simulink model "TwoTankClosedLoop"  (R2016a)
settings: Solver=ode45  StartTime=0.0  StopTime=inputOpt.simTime  MaxStep=0.2  RelTol=1e-3
undefined symbols (not defined in the file): Initials, inputOpt, kl, kv1, kv2, kv3, kv4, L1i, SPL1, SPL2, SPT1, SPT2, T1i, timeDelay
libraries: simulink x4
settings Model: Creator=blindner  LastModifiedBy=blindner
settings DataIOCC: ExternalInput=getinputstruct(op_trim1)  FinalStateName=TwoTankClosedLoopSimState  InitialState=simState  SaveFinalState=on  SaveCompleteFinalSimState=on  SaveFormat=Array  SaveOutput=off  InspectSignalLogs=on  SaveTime=off
settings DebuggingCC: SolverPrmCheckMsg=warning
settings HardwareCC: ProdBitPerPointer=32  ProdLargestAtomicFloat=None  ProdIntDivRoundTo=Undefined  ProdEndianess=Unspecified  ProdWordSize=32  ProdHWDeviceType=32-bit Generic
settings ModelReferenceCC: PropagateSignalLabelsOutOfModel=off
settings ConfigComp: CovModelRefEnable=Off  CovSFcnEnable=off

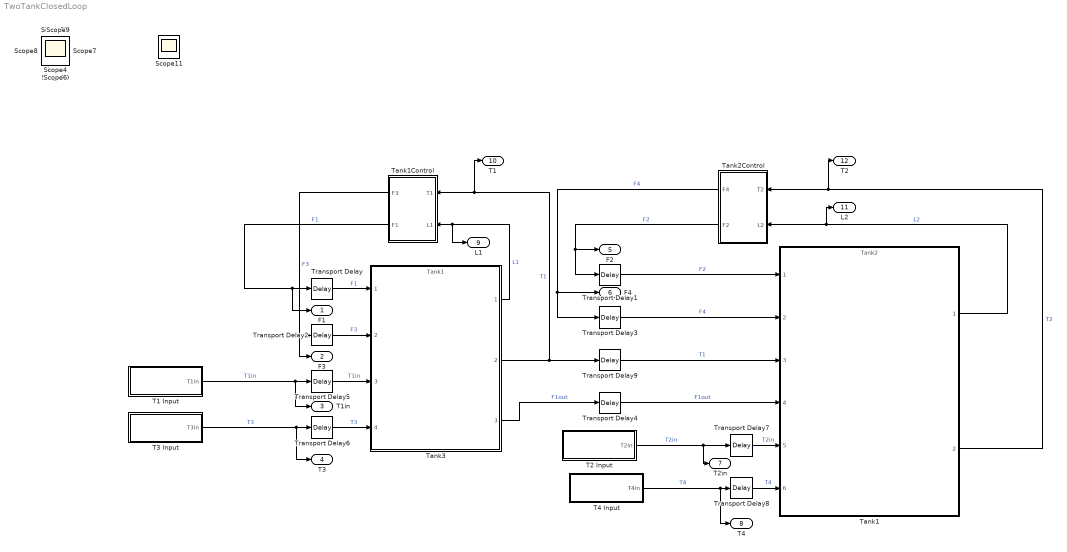
== system TwoTankClosedLoop ==
  T1 Input : Subsystem  Variant=on
  T2 Input : Subsystem  Variant=on
  T3 Input : Subsystem  Variant=on
  T4 Input : Subsystem  Variant=on
  Tank1 : ModelReference  ModelNameDialog=Tank2  SimulationMode=Normal  ModelReferenceVersion=1.153
  Tank1Control : Subsystem
  Tank2Control : Subsystem
  Tank3 : ModelReference  ModelNameDialog=Tank1  SimulationMode=Normal  ModelReferenceVersion=1.161
  Transport Delay : TransportDelay  DelayTime=timeDelay.F1  InitialOutput=Initials.F1  TransDelayFeedthrough=on
  Transport Delay1 : TransportDelay  DelayTime=timeDelay.F2  InitialOutput=Initials.F2  TransDelayFeedthrough=on
  Transport Delay2 : TransportDelay  DelayTime=timeDelay.F3  InitialOutput=Initials.F3  TransDelayFeedthrough=on
  Transport Delay3 : TransportDelay  DelayTime=timeDelay.F4  InitialOutput=Initials.F4  TransDelayFeedthrough=on
  Transport Delay4 : TransportDelay  DelayTime=timeDelay.F1Out  InitialOutput=(L1i)^0.5*kl  TransDelayFeedthrough=on
  Transport Delay5 : TransportDelay  DelayTime=timeDelay.F1  InitialOutput=inputOpt.T1in.start  TransDelayFeedthrough=on
  Transport Delay6 : TransportDelay  DelayTime=timeDelay.F3  InitialOutput=inputOpt.T3.start  TransDelayFeedthrough=on
  Transport Delay7 : TransportDelay  DelayTime=timeDelay.F2  InitialOutput=inputOpt.T2in.start  TransDelayFeedthrough=on
  Transport Delay8 : TransportDelay  DelayTime=timeDelay.F4  InitialOutput=inputOpt.T4.start  TransDelayFeedthrough=on
  Transport Delay9 : TransportDelay  DelayTime=timeDelay.F1Out  InitialOutput=T1i  TransDelayFeedthrough=on
  F1 : Outport
  F3 : Outport  Port=2
  T1in : Outport  Port=3
  T3 : Outport  Port=4
  F2 : Outport  Port=5
  F4 : Outport  Port=6
  T2in : Outport  Port=7
  T4 : Outport  Port=8
  L1 : Outport  Port=9
  T1 : Outport  Port=10
  L2 : Outport  Port=11
  T2 : Outport  Port=12
  Scope{,1..11} (12 alike) : Scope
  wires:
  Tank2Control/2(F2) -> Transport Delay1/1, F2/1  "F2"
  T2 Input/1(T2in) -> T2in/1, Transport Delay7/1  "T2in"
  Tank1/2 -> T2/1, Tank2Control/1(T2)  "T2"
  T1 Input/1(T1in) -> T1in/1, Transport Delay5/1  "T1in"
  T3 Input/1(T3in) -> T3/1, Transport Delay6/1  "T3"
  Tank1Control/2(F1) -> F1/1, Transport Delay/1  "F1"
  Tank3/3 -> Transport Delay4/1  "F1out"
  T4 Input/1(T4in) -> T4/1, Transport Delay8/1  "T4"
  Tank1Control/1(F3) -> F3/1, Transport Delay2/1  "F3"
  Tank2Control/1(F4) -> F4/1, Transport Delay3/1  "F4"
  Transport Delay5/1 -> Tank3/3  "T1in"
  Transport Delay6/1 -> Tank3/4  "T3"
  Transport Delay/1 -> Tank3/1  "F1"
  Transport Delay2/1 -> Tank3/2  "F3"
  Transport Delay3/1 -> Tank1/2  "F4"
  Transport Delay8/1 -> Tank1/6  "T4"
  Transport Delay7/1 -> Tank1/5  "T2in"
  Transport Delay9/1 -> Tank1/3  "T1"
  Transport Delay4/1 -> Tank1/4  "F1out"
  Transport Delay1/1 -> Tank1/1  "F2"
  Tank3/2 -> T1/1, Tank1Control/1(T1), Transport Delay9/1  "T1"
  Tank1/1 -> L2/1, Tank2Control/2(L2)  "L2"
  Tank3/1 -> L1/1, Tank1Control/2(L1)  "L1"

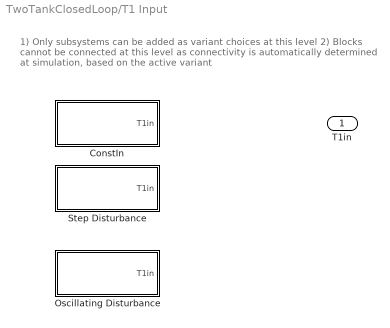
== system TwoTankClosedLoop/T1 Input ==
  note: 1) Only subsystems can be added as variant choices at this level
      | 2) Blocks cannot be connected at this level as connectivity is
      | automatically determined at simulation, based on the active variant
  ConstIn : Subsystem  VariantControl=(default)
  Oscillating Disturbance : Subsystem  VariantControl=T1Oscillating
  Step Disturbance : Subsystem  VariantControl=T1Step
  T1in : Outport

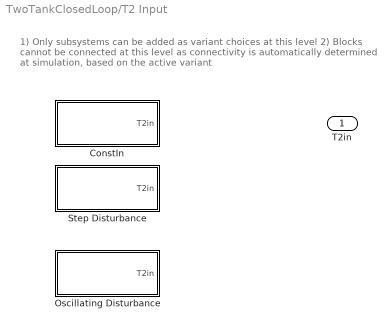
== system TwoTankClosedLoop/T2 Input ==
  note: 1) Only subsystems can be added as variant choices at this level
      | 2) Blocks cannot be connected at this level as connectivity is
      | automatically determined at simulation, based on the active variant
  ConstIn : Subsystem  VariantControl=(default)
  Oscillating Disturbance : Subsystem  VariantControl=T2Oscillating
  Step Disturbance : Subsystem  VariantControl=T2Step
  T2in : Outport

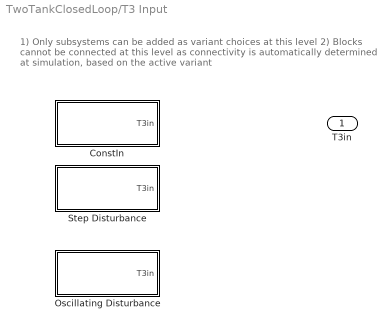
== system TwoTankClosedLoop/T3 Input ==
  note: 1) Only subsystems can be added as variant choices at this level
      | 2) Blocks cannot be connected at this level as connectivity is
      | automatically determined at simulation, based on the active variant
  ConstIn : Subsystem  VariantControl=(default)
  Oscillating Disturbance : Subsystem  VariantControl=T3Oscillating
  Step Disturbance : Subsystem  VariantControl=T3Step
  T3in : Outport

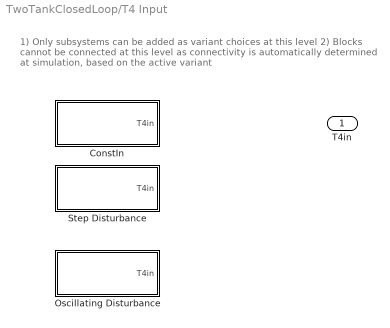
== system TwoTankClosedLoop/T4 Input ==
  note: 1) Only subsystems can be added as variant choices at this level
      | 2) Blocks cannot be connected at this level as connectivity is
      | automatically determined at simulation, based on the active variant
  ConstIn : Subsystem  VariantControl=(default)
  Oscillating Disturbance : Subsystem  VariantControl=T4Oscillating
  Step Disturbance : Subsystem  VariantControl=T4Step
  T4in : Outport

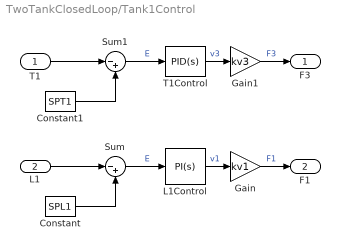
== system TwoTankClosedLoop/Tank1Control ==
  T1 : Inport
  L1 : Inport  Port=2
  Constant : Constant  Value=SPL1
  Constant1 : Constant  Value=SPT1
  Gain : Gain  Gain=kv1
  Gain1 : Gain  Gain=kv3
  L1Control : simulink/Continuous/PID Controller  Controller=PI  TimeDomain=Continuous-time  SampleTime=-1  IntegratorMethod=Forward Euler  FilterMethod=Forward Euler  Form=Parallel  UseFilter=on  ControllerParametersSource=internal  P=13  I=2  D=-46.1324731979825  N=0.0805995619975817  InitialConditionSource=internal  InitialConditionForIntegrator=Initials.F1/kv1  InitialConditionForFilter=0  ExternalReset=none  LimitOutput=on  UpperSaturationLimit=inf  LowerSaturationLimit=0  LinearizeAsGain=on  AntiWindupMode=none  Kb=1  TrackingMode=off  Kt=1  PParamMin=[]  PParamMax=[]  IParamMin=[]  IParamMax=[]  DParamMin=[]  DParamMax=[]  NParamMin=[]  NParamMax=[]  KbParamMin=[]  KbParamMax=[]  KtParamMin=[]  KtParamMax=[]  POutMin=[]  POutMax=[]  IOutMin=[]  IOutMax=[]  DOutMin=[]  DOutMax=[]  NOutMin=[]  NOutMax=[]  KbOutMin=[]  KbOutMax=[]  KtOutMin=[]  KtOutMax=[]  IntegratorOutMin=[]  IntegratorOutMax=[]  FilterOutMin=[]  FilterOutMax=[]  SumOutMin=[]  SumOutMax=[]  SumI1OutMin=[]  SumI1OutMax=[]  SumI2OutMin=[]  SumI2OutMax=[]  SumI3OutMin=[]  SumI3OutMax=[]  SumDOutMin=[]  SumDOutMax=[]  SaturationOutMin=[]  SaturationOutMax=[]  IntegratorContinuousStateAttributes=''  IntegratorStateMustResolveToSignalObject=off  IntegratorRTWStateStorageClass=Auto  FilterContinuousStateAttributes=''  FilterStateMustResolveToSignalObject=off  FilterRTWStateStorageClass=Auto  DifferentiatorICPrevScaledInput=0  DifferentiatorOutMin=[]  DifferentiatorOutMax=[]
  Sum : Sum  Inputs=|-+
  Sum1 : Sum  Inputs=|-+
  T1Control : simulink/Continuous/PID Controller  Controller=PID  TimeDomain=Continuous-time  SampleTime=-1  IntegratorMethod=Forward Euler  FilterMethod=Forward Euler  Form=Parallel  UseFilter=on  ControllerParametersSource=internal  P=9.53922380214598  I=1.41929760465604  D=0  N=100  InitialConditionSource=internal  InitialConditionForIntegrator=Initials.F3/kv3  InitialConditionForFilter=0  ExternalReset=none  LimitOutput=on  UpperSaturationLimit=inf  LowerSaturationLimit=0  LinearizeAsGain=on  AntiWindupMode=none  Kb=1  TrackingMode=off  Kt=1  PParamMin=[]  PParamMax=[]  IParamMin=[]  IParamMax=[]  DParamMin=[]  DParamMax=[]  NParamMin=[]  NParamMax=[]  KbParamMin=[]  KbParamMax=[]  KtParamMin=[]  KtParamMax=[]  POutMin=[]  POutMax=[]  IOutMin=[]  IOutMax=[]  DOutMin=[]  DOutMax=[]  NOutMin=[]  NOutMax=[]  KbOutMin=[]  KbOutMax=[]  KtOutMin=[]  KtOutMax=[]  IntegratorOutMin=[]  IntegratorOutMax=[]  FilterOutMin=[]  FilterOutMax=[]  SumOutMin=[]  SumOutMax=[]  SumI1OutMin=[]  SumI1OutMax=[]  SumI2OutMin=[]  SumI2OutMax=[]  SumI3OutMin=[]  SumI3OutMax=[]  SumDOutMin=[]  SumDOutMax=[]  SaturationOutMin=[]  SaturationOutMax=[]  IntegratorContinuousStateAttributes=''  IntegratorStateMustResolveToSignalObject=off  IntegratorRTWStateStorageClass=Auto  FilterContinuousStateAttributes=''  FilterStateMustResolveToSignalObject=off  FilterRTWStateStorageClass=Auto  DifferentiatorICPrevScaledInput=0  DifferentiatorOutMin=[]  DifferentiatorOutMax=[]
  F3 : Outport
  F1 : Outport  Port=2
  wires:
  Gain1/1 -> F3/1  "F3"
  Gain/1 -> F1/1  "F1"
  Sum1/1 -> T1Control/1  "E"
  Sum/1 -> L1Control/1  "E"
  T1Control/1 -> Gain1/1  "v3"
  L1Control/1 -> Gain/1  "v1"
  Constant1/1 -> Sum1/2
  Constant/1 -> Sum/2
  T1/1 -> Sum1/1
  L1/1 -> Sum/1

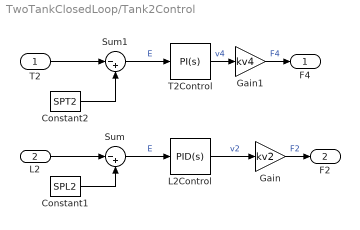
== system TwoTankClosedLoop/Tank2Control ==
  T2 : Inport
  L2 : Inport  Port=2
  Constant1 : Constant  Value=SPL2
  Constant2 : Constant  Value=SPT2
  Gain : Gain  Gain=kv2
  Gain1 : Gain  Gain=kv4
  L2Control : simulink/Continuous/PID Controller  Controller=PID  TimeDomain=Continuous-time  SampleTime=-1  IntegratorMethod=Forward Euler  FilterMethod=Forward Euler  Form=Parallel  UseFilter=on  ControllerParametersSource=internal  P=15  I=3  D=0  N=100  InitialConditionSource=internal  InitialConditionForIntegrator=Initials.F2/kv2  InitialConditionForFilter=0  ExternalReset=none  LimitOutput=on  UpperSaturationLimit=inf  LowerSaturationLimit=0  LinearizeAsGain=on  AntiWindupMode=none  Kb=1  TrackingMode=off  Kt=1  PParamMin=[]  PParamMax=[]  IParamMin=[]  IParamMax=[]  DParamMin=[]  DParamMax=[]  NParamMin=[]  NParamMax=[]  KbParamMin=[]  KbParamMax=[]  KtParamMin=[]  KtParamMax=[]  POutMin=[]  POutMax=[]  IOutMin=[]  IOutMax=[]  DOutMin=[]  DOutMax=[]  NOutMin=[]  NOutMax=[]  KbOutMin=[]  KbOutMax=[]  KtOutMin=[]  KtOutMax=[]  IntegratorOutMin=[]  IntegratorOutMax=[]  FilterOutMin=[]  FilterOutMax=[]  SumOutMin=[]  SumOutMax=[]  SumI1OutMin=[]  SumI1OutMax=[]  SumI2OutMin=[]  SumI2OutMax=[]  SumI3OutMin=[]  SumI3OutMax=[]  SumDOutMin=[]  SumDOutMax=[]  SaturationOutMin=[]  SaturationOutMax=[]  IntegratorContinuousStateAttributes=''  IntegratorStateMustResolveToSignalObject=off  IntegratorRTWStateStorageClass=Auto  FilterContinuousStateAttributes=''  FilterStateMustResolveToSignalObject=off  FilterRTWStateStorageClass=Auto  DifferentiatorICPrevScaledInput=0  DifferentiatorOutMin=[]  DifferentiatorOutMax=[]
  Sum : Sum  Inputs=|-+
  Sum1 : Sum  Inputs=|-+
  T2Control : simulink/Continuous/PID Controller  Controller=PI  TimeDomain=Continuous-time  SampleTime=-1  IntegratorMethod=Forward Euler  FilterMethod=Forward Euler  Form=Parallel  UseFilter=on  ControllerParametersSource=internal  P=5  I=0.5  D=0  N=100  InitialConditionSource=internal  InitialConditionForIntegrator=Initials.F4/kv4  InitialConditionForFilter=0  ExternalReset=none  LimitOutput=on  UpperSaturationLimit=inf  LowerSaturationLimit=0  LinearizeAsGain=on  AntiWindupMode=none  Kb=1  TrackingMode=off  Kt=1  PParamMin=[]  PParamMax=[]  IParamMin=[]  IParamMax=[]  DParamMin=[]  DParamMax=[]  NParamMin=[]  NParamMax=[]  KbParamMin=[]  KbParamMax=[]  KtParamMin=[]  KtParamMax=[]  POutMin=[]  POutMax=[]  IOutMin=[]  IOutMax=[]  DOutMin=[]  DOutMax=[]  NOutMin=[]  NOutMax=[]  KbOutMin=[]  KbOutMax=[]  KtOutMin=[]  KtOutMax=[]  IntegratorOutMin=[]  IntegratorOutMax=[]  FilterOutMin=[]  FilterOutMax=[]  SumOutMin=[]  SumOutMax=[]  SumI1OutMin=[]  SumI1OutMax=[]  SumI2OutMin=[]  SumI2OutMax=[]  SumI3OutMin=[]  SumI3OutMax=[]  SumDOutMin=[]  SumDOutMax=[]  SaturationOutMin=[]  SaturationOutMax=[]  IntegratorContinuousStateAttributes=''  IntegratorStateMustResolveToSignalObject=off  IntegratorRTWStateStorageClass=Auto  FilterContinuousStateAttributes=''  FilterStateMustResolveToSignalObject=off  FilterRTWStateStorageClass=Auto  DifferentiatorICPrevScaledInput=0  DifferentiatorOutMin=[]  DifferentiatorOutMax=[]
  F4 : Outport
  F2 : Outport  Port=2
  wires:
  Gain1/1 -> F4/1  "F4"
  Gain/1 -> F2/1  "F2"
  Sum1/1 -> T2Control/1  "E"
  Sum/1 -> L2Control/1  "E"
  Constant1/1 -> Sum/2
  Constant2/1 -> Sum1/2
  L2Control/1 -> Gain/1  "v2"
  T2Control/1 -> Gain1/1  "v4"
  T2/1 -> Sum1/1
  L2/1 -> Sum/1

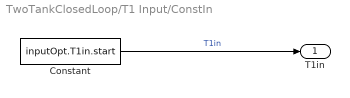
== system TwoTankClosedLoop/T1 Input/ConstIn ==
  Constant : Constant  Value=inputOpt.T1in.start
  T1in : Outport
  wires:
  Constant/1 -> T1in/1  "T1in"

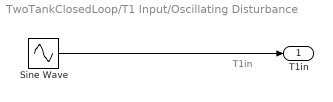
== system TwoTankClosedLoop/T1 Input/Oscillating Disturbance ==
  note: T1in
  Sine Wave : Sin  Amplitude=inputOpt.T1in.amplitude  Bias=inputOpt.T1in.start  Frequency=pi/inputOpt.T1in.period  SampleTime=0
  T1in : Outport
  wires:
  Sine Wave/1 -> T1in/1

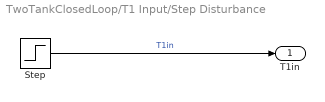
== system TwoTankClosedLoop/T1 Input/Step Disturbance ==
  Step : Step  Time=inputOpt.T1in.time  Before=inputOpt.T1in.start  After=inputOpt.T1in.end  SampleTime=0
  T1in : Outport
  wires:
  Step/1 -> T1in/1  "T1in"

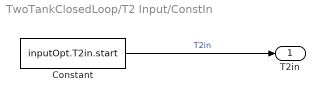
== system TwoTankClosedLoop/T2 Input/ConstIn ==
  Constant : Constant  Value=inputOpt.T2in.start
  T2in : Outport
  wires:
  Constant/1 -> T2in/1  "T2in"

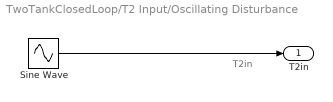
== system TwoTankClosedLoop/T2 Input/Oscillating Disturbance ==
  note: T2in
  Sine Wave : Sin  Amplitude=inputOpt.T2in.amplitude  Bias=inputOpt.T2in.start  Frequency=pi/inputOpt.T2in.amplitude  SampleTime=0
  T2in : Outport
  wires:
  Sine Wave/1 -> T2in/1

== system TwoTankClosedLoop/T2 Input/Step Disturbance ==
  Step : Step  Time=inputOpt.T2in.time  Before=inputOpt.T2in.start  After=inputOpt.T2in.end  SampleTime=0
  T2in : Outport
  wires:
  Step/1 -> T2in/1  "T2in"

== system TwoTankClosedLoop/T3 Input/ConstIn ==
  Constant : Constant  Value=inputOpt.T3.start
  T3in : Outport
  wires:
  Constant/1 -> T3in/1  "T3in"

== system TwoTankClosedLoop/T3 Input/Oscillating Disturbance ==
  note: T3in
  Sine Wave : Sin  Amplitude=inputOpt.T3.amplitude  Bias=inputOpt.T3.start  Frequency=pi/inputOpt.T3.period  SampleTime=0
  T3in : Outport
  wires:
  Sine Wave/1 -> T3in/1

== system TwoTankClosedLoop/T3 Input/Step Disturbance ==
  Step : Step  Time=inputOpt.T3.time  Before=inputOpt.T3.start  After=inputOpt.T3.end  SampleTime=0
  T3in : Outport
  wires:
  Step/1 -> T3in/1  "T3in"

== system TwoTankClosedLoop/T4 Input/ConstIn ==
  Constant : Constant  Value=inputOpt.T4.start
  T4in : Outport
  wires:
  Constant/1 -> T4in/1  "T3in"

== system TwoTankClosedLoop/T4 Input/Oscillating Disturbance ==
  note: T4in
  Sine Wave : Sin  Amplitude=inputOpt.T4.amplitude  Bias=inputOpt.T4.start  Frequency=pi/inputOpt.T4.period  SampleTime=0
  T4in : Outport
  wires:
  Sine Wave/1 -> T4in/1

== system TwoTankClosedLoop/T4 Input/Step Disturbance ==
  Step : Step  Time=inputOpt.T4.time  Before=inputOpt.T4.start  After=inputOpt.T4.end  SampleTime=0
  T4in : Outport
  wires:
  Step/1 -> T4in/1  "T4in"
